simulink model "LQR"  (R2022a)
settings: Solver=ode4  StartTime=0.0  StopTime=SIM_TIME  FixedStep=STEP_SIZE  RelTol=1e-3
values from neighbouring files (symbols this model uses):
  bc = 2    [ode1.m]
  bp = 0.1    [ode1.m]
undefined symbols (not defined in the file or in its folder): bm, g, Jm, Jp, ke, kt, l, Lm, m, M, r, Rm, theta0, theta_dot0, x0, x_dot0
settings Model: Creator=farfar  LastModifiedBy=farfar
settings DataIOCC: ExternalInput=[0, 0]  InitialState=[]  LoadExternalInput=on  LoadInitialState=on  ReturnWorkspaceOutputs=off

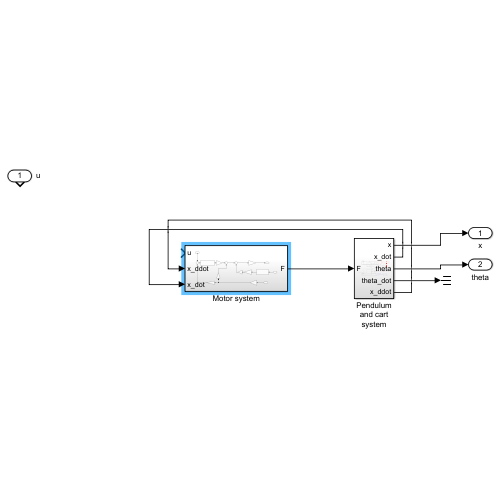
[thumbnail: Simulink's stored preview of the top-level diagram]
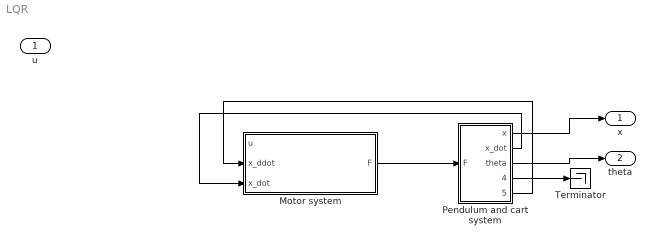
== system LQR ==
  u : Inport
  Motor system : Subsystem
  Pendulum and cart system : Subsystem
  Terminator : Terminator
  x : Outport
  theta : Outport  Port=2
  wires:
  Pendulum and cart system/5(x_ddot) -> Motor system/2(x_ddot)
  Pendulum and cart system/2(x_dot) -> Motor system/3(x_dot)
  Pendulum and cart system/4(theta_dot) -> Terminator/1
  Pendulum and cart system/1(x) -> x/1
  Pendulum and cart system/3(theta) -> theta/1
  Motor system/1(F) -> Pendulum and cart system/1(F)

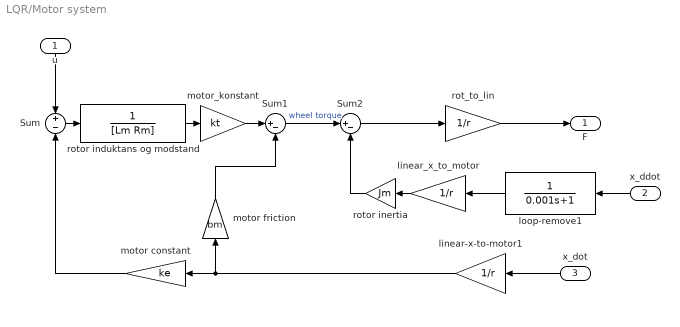
== system LQR/Motor system ==
  u : Inport
  x_ddot : Inport  Port=2
  x_dot : Inport  Port=3
  Sum : Sum  Inputs=+|-
  Sum1 : Sum  Inputs=|+-
  Sum2 : Sum  Inputs=|+-
  linear-x-to-motor1 : Gain  Gain=1/r
  linear_x_to_motor : Gain  Gain=1/r
  loop-remove1 : TransferFcn  Denominator=[0.001 1]
  motor constant : Gain  Gain=ke
  motor friction : Gain  Gain=bm
  motor_konstant : Gain  Gain=kt
  rot_to_lin : Gain  Gain=1/r
  rotor induktans og modstand : TransferFcn  Denominator=[Lm Rm]
  rotor inertia : Gain  Gain=Jm
  F : Outport
  wires:
  linear-x-to-motor1/1 -> motor constant/1, motor friction/1
  rotor induktans og modstand/1 -> motor_konstant/1
  u/1 -> Sum/1
  linear_x_to_motor/1 -> rotor inertia/1
  Sum2/1 -> rot_to_lin/1
  x_dot/1 -> linear-x-to-motor1/1
  rot_to_lin/1 -> F/1
  x_ddot/1 -> loop-remove1/1
  Sum/1 -> rotor induktans og modstand/1
  motor constant/1 -> Sum/2
  Sum1/1 -> Sum2/1  "wheel torque"
  rotor inertia/1 -> Sum2/2
  motor friction/1 -> Sum1/2
  motor_konstant/1 -> Sum1/1
  loop-remove1/1 -> linear_x_to_motor/1

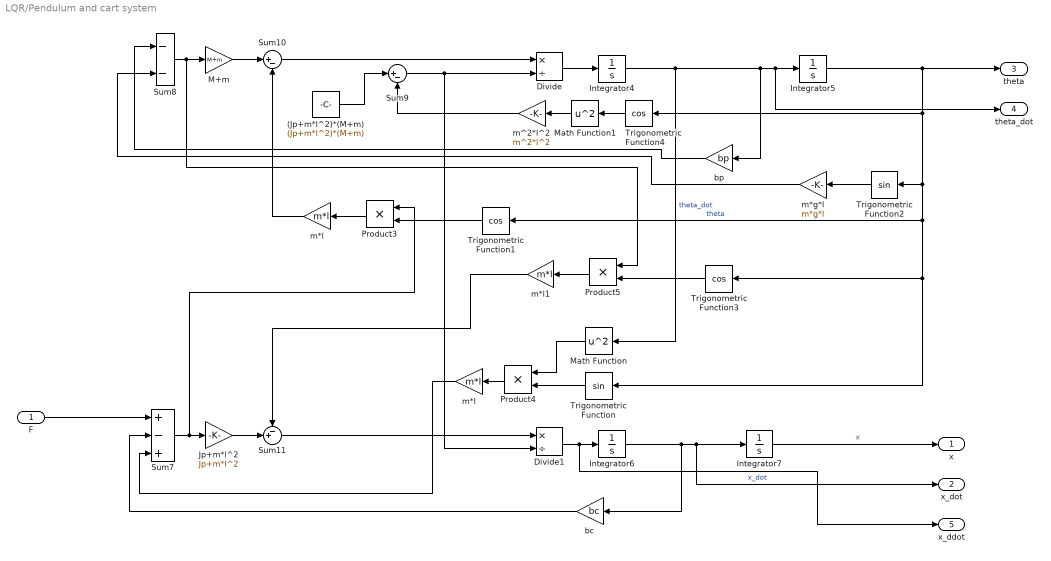
== system LQR/Pendulum and cart system ==
  F : Inport
  (Jp+m*l^2)*(M+m) : Constant  Value=(Jp+m*l^2)*(M+m)
  Divide : Product  Inputs=*/
  Divide1 : Product  Inputs=*/
  Integrator4 : Integrator  Priority=1  InitialCondition=theta_dot0  ContinuousStateAttributes='pendulum.angular.velocity'
  Integrator5 : Integrator  Priority=2  InitialCondition=theta0  UpperSaturationLimit=pi  LowerSaturationLimit=-pi  ContinuousStateAttributes='pendulum.angular.position'
  Integrator6 : Integrator  Priority=3  InitialCondition=x_dot0  ContinuousStateAttributes='trolley.horizontal.velocity'
  Integrator7 : Integrator  Priority=4  InitialCondition=x0  ContinuousStateAttributes='trolley.horizontal.position'
  Jp+m*l^2 : Gain  Gain=Jp+m*l^2
  M+m : Gain  Gain=M+m
  Math Function : Math  Operator=square  SignedPower=on
  Math Function1 : Math  Operator=square  SignedPower=on
  Product3 : Product
  Product4 : Product
  Product5 : Product
  Sum10 : Sum  Inputs=|+-
  Sum11 : Sum  Inputs=-+|
  Sum7 : Sum  Inputs=+-+
  Sum8 : Sum  Inputs=--
  Sum9 : Sum  Inputs=|+-
  Trigonometric Function : Trigonometry
  Trigonometric Function1 : Trigonometry  Operator=cos
  Trigonometric Function2 : Trigonometry
  Trigonometric Function3 : Trigonometry  Operator=cos
  Trigonometric Function4 : Trigonometry  Operator=cos
  bc : Gain  Gain=bc
  bp : Gain  Gain=bp
  m*g*l : Gain  Gain=m*g*l
  m*l : Gain  Gain=m*l
  "m*l " : Gain  Gain=m*l
  m*l1 : Gain  Gain=m*l
  m^2*l^2 : Gain  Gain=m^2*l^2
  x : Outport
  x_dot : Outport  Port=2
  theta : Outport  Port=3
  theta_dot : Outport  Port=4
  x_ddot : Outport  Port=5
  wires:
  Integrator6/1 -> bc/1, x_dot/1, Integrator7/1  "x_dot"
  Integrator4/1 -> Math Function/1, bp/1, theta_dot/1, Integrator5/1  "theta_dot"
  Math Function1/1 -> m^2*l^2/1
  M+m/1 -> Sum10/1
  Math Function/1 -> Product4/1
  Sum10/1 -> Divide/1
  Trigonometric Function4/1 -> Math Function1/1
  Product4/1 -> "m*l "/1
  Jp+m*l^2/1 -> Sum11/2
  Trigonometric Function/1 -> Product4/2
  m*l1/1 -> Sum11/1
  Integrator5/1 -> theta/1, Trigonometric Function4/1, Trigonometric Function2/1, Trigonometric Function1/1, Trigonometric Function3/1, Trigonometric Function/1  "theta"
  Sum7/1 -> Product3/1, Jp+m*l^2/1
  m*g*l/1 -> Sum8/2
  Sum9/1 -> Divide1/2, Divide/2
  Integrator7/1 -> x/1  "x"
  Divide/1 -> Integrator4/1
  Trigonometric Function2/1 -> m*g*l/1
  "m*l "/1 -> Sum7/3
  Trigonometric Function1/1 -> Product3/2
  Divide1/1 -> x_ddot/1, Integrator6/1
  bc/1 -> Sum7/2
  bp/1 -> Sum8/1
  Product3/1 -> m*l/1
  (Jp+m*l^2)*(M+m)/1 -> Sum9/1
  Sum8/1 -> Product5/1, M+m/1
  m^2*l^2/1 -> Sum9/2
  Sum11/1 -> Divide1/1
  m*l/1 -> Sum10/2
  Product5/1 -> m*l1/1
  Trigonometric Function3/1 -> Product5/2
  F/1 -> Sum7/1
